simulink model "hm3_closed_loop"  (R2025b)
settings: Solver=ode45  StartTime=0.0  StopTime=Tstop  RelTol=1e-3
undefined symbols (not defined in the file): A_full, A_rigid, Bdelta_full, Bdelta_rigid, Bwind_full, Bwind_rigid, C_meas_full, C_meas_rigid, C_plot_full, C_plot_rigid, Kd_th, Kd_z, Kp_th, Kp_z, notch_den, notch_num, tvc_den, tvc_num
settings Model: Creator=nickd  LastModifiedBy=nickd

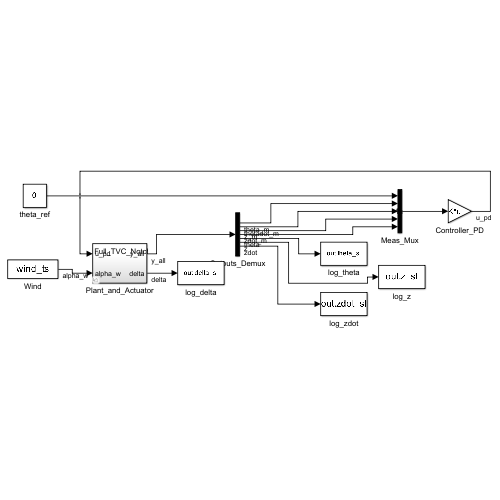
[thumbnail: Simulink's stored preview of the top-level diagram]
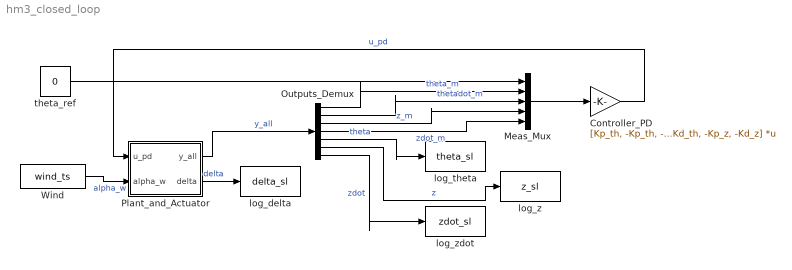
== system hm3_closed_loop ==
  Controller_PD : Gain  Gain=[Kp_th, -Kp_th, -Kd_th, -Kp_z, -Kd_z]  Multiplication=Matrix(K*u)
  Meas_Mux : Mux  Inputs=5
  Outputs_Demux : Demux  Outputs=7
  Plant_and_Actuator : Subsystem  Variant=on
  Wind : FromWorkspace  VariableName=wind_ts  OutputAfterFinalValue=Holding final value
  log_delta : ToWorkspace  VariableName=delta_sl  SaveFormat=Timeseries  SampleTime=-1
  log_theta : ToWorkspace  VariableName=theta_sl  SaveFormat=Timeseries  SampleTime=-1
  log_z : ToWorkspace  VariableName=z_sl  SaveFormat=Timeseries  SampleTime=-1
  log_zdot : ToWorkspace  VariableName=zdot_sl  SaveFormat=Timeseries  SampleTime=-1
  theta_ref : Constant  Value=0
  wires:
  Outputs_Demux/7 -> log_zdot/1  "zdot"
  Outputs_Demux/6 -> log_z/1  "z"
  Outputs_Demux/5 -> log_theta/1  "theta"
  Outputs_Demux/4 -> Meas_Mux/5  "zdot_m"
  Outputs_Demux/3 -> Meas_Mux/4  "z_m"
  Outputs_Demux/2 -> Meas_Mux/3  "thetadot_m"
  Outputs_Demux/1 -> Meas_Mux/2  "theta_m"
  Meas_Mux/1 -> Controller_PD/1
  theta_ref/1 -> Meas_Mux/1
  Controller_PD/1 -> Plant_and_Actuator/1(u_pd)  "u_pd"
  Wind/1 -> Plant_and_Actuator/2(alpha_w)  "alpha_w"
  Plant_and_Actuator/1(y_all) -> Outputs_Demux/1  "y_all"
  Plant_and_Actuator/2(delta) -> log_delta/1  "delta"

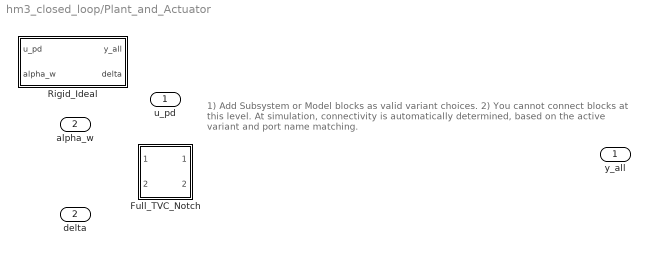
== system hm3_closed_loop/Plant_and_Actuator ==
  note: 1) Add Subsystem or Model blocks as valid variant choices.
      | 2) You cannot connect blocks at this level. At simulation, connectivity is automatically
      | determined, based on the active variant and port name matching.
  u_pd : Inport
  alpha_w : Inport  Port=2
  Full_TVC_Notch : Subsystem  VariantControl=task ~= 1
  Rigid_Ideal : Subsystem  VariantControl=task == 1
  y_all : Outport
  delta : Outport  Port=2

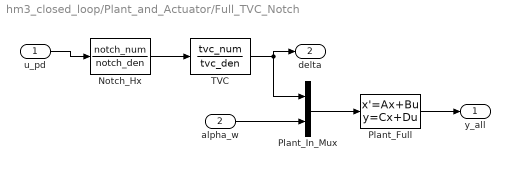
== system hm3_closed_loop/Plant_and_Actuator/Full_TVC_Notch ==
  u_pd : Inport
  alpha_w : Inport  Port=2
  Notch_Hx : TransferFcn  Numerator=notch_num  Denominator=notch_den
  Plant_Full : StateSpace  A=A_full  B=[Bdelta_full, Bwind_full]  C=[C_meas_full; C_plot_full]  D=zeros(7,2)
  Plant_In_Mux : Mux  Inputs=2
  TVC : TransferFcn  Numerator=tvc_num  Denominator=tvc_den
  y_all : Outport
  delta : Outport  Port=2
  wires:
  Plant_Full/1 -> y_all/1
  Plant_In_Mux/1 -> Plant_Full/1
  alpha_w/1 -> Plant_In_Mux/2
  TVC/1 -> Plant_In_Mux/1, delta/1
  Notch_Hx/1 -> TVC/1
  u_pd/1 -> Notch_Hx/1

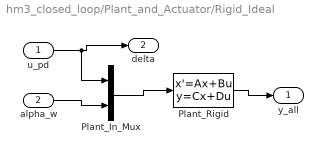
== system hm3_closed_loop/Plant_and_Actuator/Rigid_Ideal ==
  u_pd : Inport
  alpha_w : Inport  Port=2
  Plant_In_Mux : Mux  Inputs=2
  Plant_Rigid : StateSpace  A=A_rigid  B=[Bdelta_rigid, Bwind_rigid]  C=[C_meas_rigid; C_plot_rigid]  D=zeros(7,2)
  y_all : Outport
  delta : Outport  Port=2
  wires:
  u_pd/1 -> delta/1, Plant_In_Mux/1
  alpha_w/1 -> Plant_In_Mux/2
  Plant_In_Mux/1 -> Plant_Rigid/1
  Plant_Rigid/1 -> y_all/1
